simulink model "STM32_matlab_communication_test"  (R2023b)
settings: Solver=VariableStepAuto  StartTime=0.0  StopTime=inf  RelTol=1e-3
libraries: instrumentseriallib x3, sldrtlib x1
settings Model: Creator=Badda_Bing  LastModifiedBy=Badda_Bing

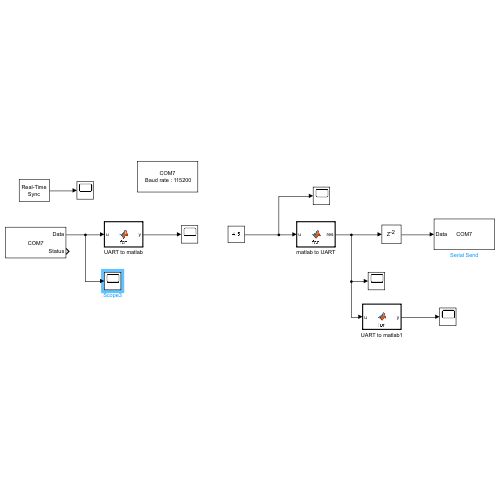
[thumbnail: Simulink's stored preview of the top-level diagram]
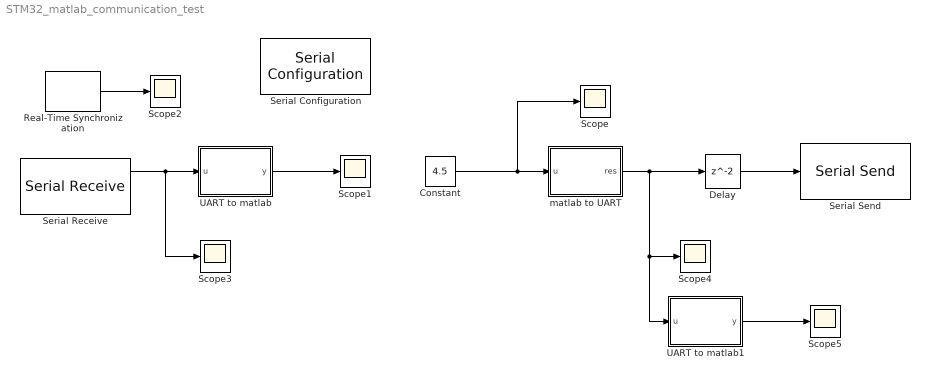
== system STM32_matlab_communication_test ==
  Constant : Constant  Value=4.5
  Delay : Delay
  Real-Time Synchronization : sldrtlib/Real-Time Synchronization  SampleTime=0.01  MaxMissedTicks=inf  ShowMissedTicks=on  YieldWhenWaiting=off
  Scope{,1..5} (6 alike) : Scope
  Serial Configuration : instrumentseriallib/Serial Configuration  Priority=-200000  PortSel=COM7  Port=COM7  ComPort=COM7  BaudRate=115200  DataBits=8  Parity=none  StopBits=1  ByteOrder=little-endian  FlowControl=none  Timeout=10  SimulateUsing=Interpreted execution  BlockInModel=on  aMode=1
      settings: LibrarySourceBlock=embeddedtargetslib/Host Communication/Serial Configuration
  Serial Receive : instrumentseriallib/Serial Receive  Priority=1  PortSel=COM7  Port=COM7  ComPort=COM7  DataType=uint8  SaveDataType=uint8  ToggleHeader=off  Header=[]  ToggleTerminator=off  Terminator=<none>  CustomTerminator=[]  InputFormat=Column major  ToggleDataSize=on  DataSize=[1 8]  EnableBlockingMode=off  ActionDataUnavailable=Output last received value  ActionWhenDataUnavailable=Output last received value  CustomValue=0  SampleTime=0.01  SimulateUsing=Interpreted execution  BlockInModel=on  aMode=1
      settings: LibrarySourceBlock=embeddedtargetslib/Host Communication/Serial Receive
  Serial Send : instrumentseriallib/Serial Send  Priority=1  PortSel=COM7  Port=COM7  ComPort=COM7  Header=[]  Terminator=<none>  CustomTerminator=[]  EnableBlockingMode=off  SimulateUsing=Interpreted execution  BlockInModel=on  aMode=1
      settings: LibrarySourceBlock=embeddedtargetslib/Host Communication/Serial Send
  UART to matlab : MATLAB Function  TreatAsAtomicUnit=on
  UART to matlab1 : MATLAB Function  TreatAsAtomicUnit=on
  matlab to UART : MATLAB Function  TreatAsAtomicUnit=on
  wires:
  Real-Time Synchronization/1 -> Scope2/1
  matlab to UART/1(res) -> Delay/1, UART to matlab1/1(u), Scope4/1
  Constant/1 -> Scope/1, matlab to UART/1(u)
  UART to matlab/1(y) -> Scope1/1
  Serial Receive/1 -> UART to matlab/1(u), Scope3/1
  UART to matlab1/1(y) -> Scope5/1
  Delay/1 -> Serial Send/1

== matlab function STM32_matlab_communication_test/matlab to UART ==
  data: u input double; res output uint8 size=[1,8]
function res = fcn(u)
    % If it is a noninteger => convert to float.
temp = cast(u,"single");
temp = typecast(temp, "uint8");

res = [1, 0, 0, 0, temp];

== matlab function STM32_matlab_communication_test/UART to matlab1 ==
  data: u input uint8 size=[1,8]; y output single
function y = fcn(u)
    temp1 = u(5:8);
    temp = typecast(temp1,"single");
y = temp;

== matlab function STM32_matlab_communication_test/UART to matlab ==
  data: u input uint8 size=[1,8]; y output single
function y = fcn(u)
    temp1 = u(5:8);
    temp = typecast(temp1,"single");
y = temp;
